simulink model "RLC"  (R2021b)
settings: Solver=VariableStepAuto  StartTime=0  StopTime=0.055  RelTol=1e-3
settings Model: Creator=juandiegocastropadilla  LastModifiedBy=juandiegocastropadilla

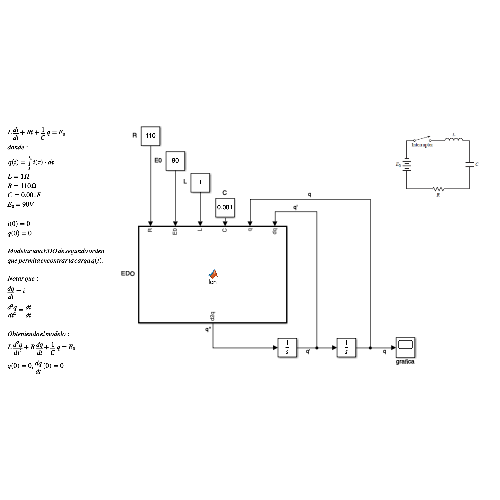
[thumbnail: Simulink's stored preview of the top-level diagram]
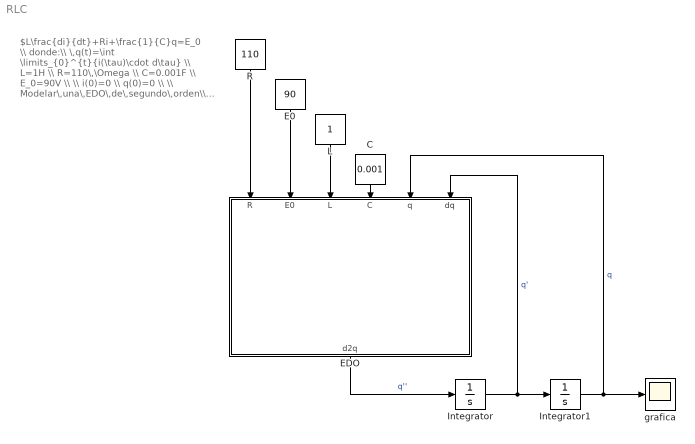
== system RLC ==
  note: $L\frac{di}{dt}+Ri+\frac{1}{C}q=E_0 \\ donde:\\ \,q(t)=\int \limits_{0}^{t}{i(\tau)\cdot d\tau} \\ L=1H \\ R=110\,\Omega \\ C=0.001F \\ E_0=90V \\ \\ i(0)=0 \\ q(0)=0 \\ \\ Modelar\,una\,EDO\,de\,segundo\,orden\\ que\,permita\,encontrar\,la\,carga\,q(t). \\ \\ Notar\,que: \\ \frac{dq}{dt}=i \\ \frac{d^2q}{dt^2}=\frac{di}{dt} \\ \\ Obteniendo\,el\,modelo: \\ L\frac{d^2q}{dt^2}+R\frac{dq}{dt}+\frac{1}{C}q=E_0 \\ q(0)=0,\,\frac{dq}{dt}(0)=0$
  " EDO" : MATLAB Function  TreatAsAtomicUnit=on
  C : Constant  Value=0.001
  E0 : Constant  Value=90
  Integrator : Integrator
  Integrator1 : Integrator
  L : Constant
  R : Constant  Value=110
  grafica : Scope
  wires:
  Integrator/1 -> Integrator1/1, " EDO"/6(dq)  "q'"
  " EDO"/1(d2q) -> Integrator/1  "q''"
  R/1 -> " EDO"/1(R)
  E0/1 -> " EDO"/2(E0)
  L/1 -> " EDO"/3(L)
  C/1 -> " EDO"/4(C)
  Integrator1/1 -> grafica/1, " EDO"/5(q)  "q"

== matlab function RLC/ EDO ==
  data: R input; E0 input; L input; C input; d2q output; q input; dq input
function d2q = fcn(R, E0, L, C, q, dq)
%#codegen

d2q = (E0-(1/C)*q-R*dq)/L;
